simulink model "CamTest_D02"  (R2018b)
settings: Solver=ode3  StartTime=0.0  StopTime=30  RelTol=1e-3  EnableMultiTasking=on
libraries: embdlinuxlib x2
settings Model: FPTRunName=Active  SimulationMode=external  ExtModeTrigDuration=2  Creator=Amir  LastModifiedBy=Amir
settings SolverCC: PositivePriorityOrder=on
settings DataIOCC: LimitDataPoints=on  SaveFormat=Array
settings OptimizationCC: ExpressionDepthLimit=2147483647  LifeSpan=Inf  MaxStackSize=64
settings DebuggingCC: UnderspecifiedInitializationDetection=Classic  MergeDetectMultiDrivingBlocksExec=none  FcnCallInpInsideContextMsg=warning  AllowSymbolicDim=off  StateNameClashWarn=warning  SFUnexpectedBacktrackingDiag=warning  SFNoUnconditionalDefaultTransitionDiag=warning  SFExecutionAtInitializationDiag=none
settings HardwareCC: ProdBitPerPointer=32  ProdBitPerSizeT=32  ProdBitPerPtrDiffT=32  ProdLargestAtomicInteger=Long  ProdLargestAtomicFloat=Double  ProdWordSize=32  ProdHWDeviceType=ARM Compatible->ARM Cortex  UseEmbeddedCoderFeatures=off
settings ModelReferenceCC: PropagateSignalLabelsOutOfModel=off
settings SFSimCC: SimUseLocalCustomCode=off
settings RTWCC: SystemTargetFile=ert.tlc  HardwareBoard=Raspberry Pi  TemplateMakefile=ert_default_tmf  GenerateReport=on  RTWVerbose=off  RTWUseLocalCustomCode=off  Toolchain=GNU GCC Raspberry Pi  BuildConfiguration=Faster Runs  LaunchReport=on
settings CodeAppCC: ForceParamTrailComments=on  OperatorAnnotations=on  StateflowObjectComments=on  MATLABSourceComments=on
settings ERTTargetCC: MultiwordLength=2048  ERTCustomFileBanners=off  SupportContinuousTime=on  SupportNonInlinedSFcns=on  RemoveResetFunc=off  SupportVariableSizeSignals=on  ModelStepFunctionPrototypeControlCompliant=off
settings ConfigComp: CovMetricSettings=dw  CovHtmlReporting=on  CovSaveCumulativeToWorkspaceVar=on  CovSaveSingleToWorkspaceVar=on  CovExternalEMLEnable=off  CovSFcnEnable=off

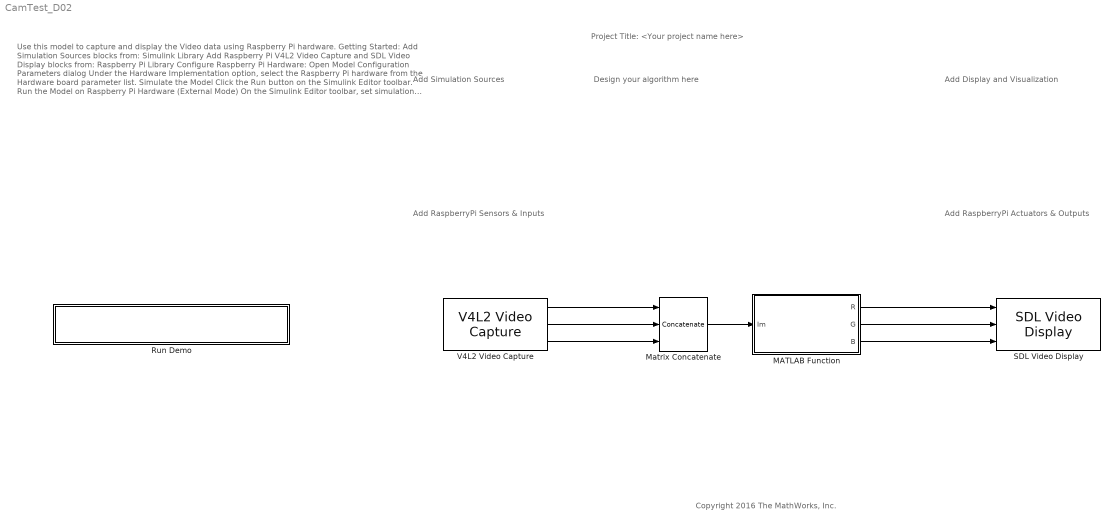
== system CamTest_D02 ==
  note: Use this model to capture and display the Video data using Raspberry Pi hardware.
      |
      | Getting Started:
      |
      | Add Simulation Sources blocks from:
      | Simulink Library
      | Add Raspberry Pi V4L2 Video Capture and SDL Video Display blocks from:
      | Raspberry Pi Library
      |
      | Configure Raspberry Pi Hardware:
      |
      | Open Model Configuration Parameters dialog
      | Under the Hardware Implementation option, select the Raspberry Pi hardware from the Hardware board parameter list.
      |
      | Simulate the Model
      |
      | Click the Run button on the Simulink Editor toolbar.
      |
      | Run the Model on Raspberry Pi Hardware (External Mode)
      |
      | On the Simulink Editor toolbar, set simulation mode to External
      |
      | External mode will stop when the number of seconds specified in the Simulation stop time parameter elapses.
      |
      | Learn More
      |
      | V4L2 Video Capture
      |
      | SDL Video Display
  note: Add RaspberryPi Sensors & Inputs
  note: Add Display and Visualization
  note: Project Title: <Your project name here>
  note: Add RaspberryPi Actuators & Outputs
  note: Add Simulation Sources
  note: Copyright 2016 The MathWorks, Inc.
  note: Design your algorithm here
  MATLAB Function : MATLAB Function  TreatAsAtomicUnit=on
  Matrix Concatenate : Concatenate  NumInputs=3  Mode=Multidimensional array  ConcatenateDimension=3
  Run Demo : Subsystem  Description=Controls host-side RTDX processing.
      mask Display: pic=imread('raspberrypiExternalMode.png');image(pic);
  SDL Video Display : embdlinuxlib/SDL Video Display  pixelFormat=RGB  pixelOrder=Planar  rowMajor=on  blockPlatform=Raspberry Pi
      settings: SourceProductName=Simulink Support Package for Raspberry Pi Hardware  SourceProductBaseCode=RASPPI
  V4L2 Video Capture : embdlinuxlib/V4L2 Video Capture  m_devName='/dev/video0'  roi=[0, 0, 640, 480]  imSizeSelection=320x240  imSize=[640, 480]  pixelFormat=RGB  pixelOrder=Planar  sampleTime=1/20  simOutput=Colorbars  blockPlatform=Raspberry Pi
      settings: SourceProductName=Simulink Support Package for Raspberry Pi Hardware  SourceProductBaseCode=RASPPI
  wires:
  Matrix Concatenate/1 -> MATLAB Function/1(Im)
  V4L2 Video Capture/1 -> Matrix Concatenate/1
  V4L2 Video Capture/2 -> Matrix Concatenate/2
  V4L2 Video Capture/3 -> Matrix Concatenate/3
  MATLAB Function/2(G) -> SDL Video Display/2
  MATLAB Function/1(R) -> SDL Video Display/1
  MATLAB Function/3(B) -> SDL Video Display/3

== system CamTest_D02/Run Demo ==

== matlab function CamTest_D02/MATLAB Function ==
  data: Im input; R output; G output; B output
function [R,G,B] = fcn(Im)
[m,n,~]=size(Im);
mask=zeros(m,n);
Im_HSV = rgb2hsv(Im);
R_T=115;%[115 135]
S_T=55;%[55 65]
for i=1:m
    for j=1:n
        if Im(i,j,1)>=R_T
            if Im(i,j,1)>=Im(i,j,2) && Im(i,j,2)>=Im(i,j,3)
                if Im_HSV(i,j,2)>=(255-Im(i,j,1))*S_T/R_T
                    mask(i,j)=1;
                end
            end
        end
    end
end
Im1= bsxfun(@times, Im, cast(mask, 'like', Im));
R=Im1(:,:,1);
G=Im1(:,:,2);
B=Im1(:,:,3);
